simulink model "Discrete_Domain"  (R2020a)
settings: Solver=VariableStepAuto  StartTime=0.0  StopTime=20  RelTol=1e-3
libraries: cstblocks x18
settings Model: Creator=Tayla  LastModifiedBy=Tayla
settings SolverCC: AlgebraicLoopSolver=LineSearch
settings DebuggingCC: AlgebraicLoopMsg=none
settings ConfigComp: PLC_TargetIDE=codesys23

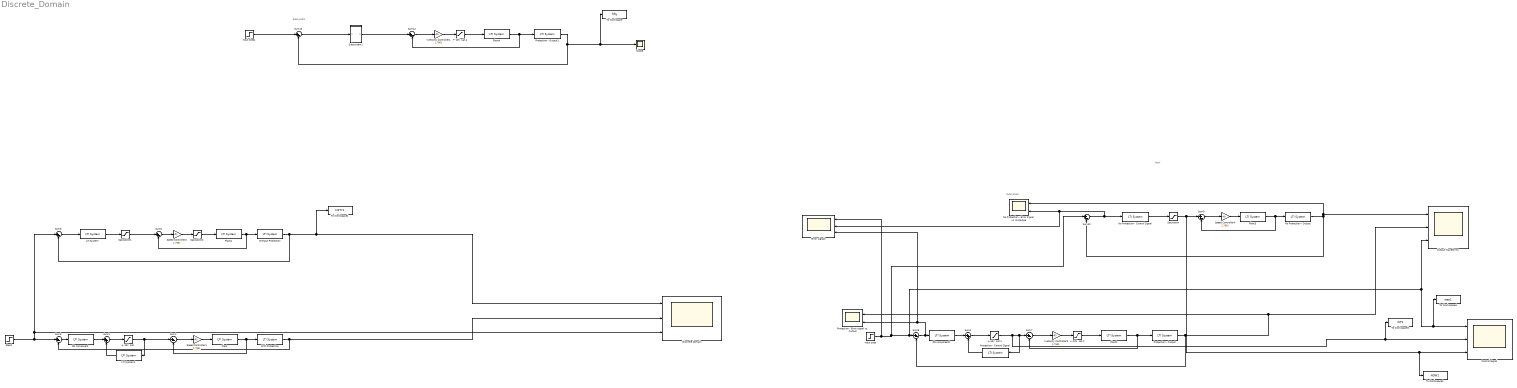
== system Discrete_Domain ==
  note: NoW
  note: Subsystem
  note: Subsystem
  " Protection - Output" : cstblocks/LTI System  sys=effectsD  IC=[]
  " Protection - Output1" : cstblocks/LTI System  sys=effectsD  IC=[]
  +-10V  sat.{,1..2,4} (4 alike) : Saturate  UpperLimit=10  LowerLimit=-10  LinearizeAsGain=off  ZeroCross=off
  Control Signal : Scope  NumInputPorts=3
  Discrete Domain : Scope  NumInputPorts=3
  Error signals : Scope  NumInputPorts=3
  Input step : Step  Time=0  After=2.61  SampleTime=0
  Input step1 : Step  After=4.35  SampleTime=0
  LTI System : cstblocks/LTI System  sys=Pos_HPF_2_Dis  IC=[]
  LTI System1 : cstblocks/LTI System  sys=PI_Dis  IC=[]
  No Protection - Control Signal : cstblocks/LTI System  sys=Pos_HPF_2_Dis  IC=[]
  No Protection - Error signal vs. Outputpe : Scope  NumInputPorts=2
  No Protection - Output : cstblocks/LTI System  sys=effectsD  IC=[]
  Output Waveforms : Scope  NumInputPorts=3
  PD component : cstblocks/LTI System  sys=Kp_Dis  IC=[]
  PD component1 : cstblocks/LTI System  sys=Kp_Dis  IC=[]
  Plant : cstblocks/LTI System  sys=tf_2  IC=[]
  Plant{1..4} (4 alike) : cstblocks/LTI System  sys=tf_1  IC=[]
  Protection - Control Signal : cstblocks/LTI System  sys=PI_Dis  IC=[]
  Protection - Error signal vs. Output : Scope  NumInputPorts=2
  Saturation : Saturate  UpperLimit=10  LowerLimit=-10
  Saturation1 : Saturate  UpperLimit=10  LowerLimit=-10
  Saturation2 : Saturate  UpperLimit=10  LowerLimit=-10
  Scope : Scope
  Speed Controller1 : Gain  Gain=1.7961
  Speed Controller2 : Gain  Gain=1.7961
  Speed Controller4 : Gain  Gain=1.7961
  Step1 : Step  After=4.35  SampleTime=0.15
  Subsystem1 : Subsystem  TreatAsAtomicUnit=on  SystemSampleTime=0.15
  Sum1 : Sum  Inputs=|++
  Sum{2..3,5..10,12..13} (10 alike) : Sum  Inputs=|+-
  Sum4 : Sum  Inputs=|++
  To Workspace : ToWorkspace  VariableName=fifty  SaveFormat=Timeseries  SampleTime=0.15
  To Workspace1 : ToWorkspace  VariableName=FIFTY1  SaveFormat=Timeseries  SampleTime=-1
  To Workspace2 : ToWorkspace  VariableName=NOW1  SaveFormat=Timeseries  SampleTime=0.15
  To Workspace3 : ToWorkspace  VariableName=WP1  SaveFormat=Timeseries  SampleTime=0.15
  To Workspace4 : ToWorkspace  VariableName=step1  SaveFormat=Timeseries  SampleTime=0.15
  Vvelocity Controller1 : Gain  Gain=1.7961
  Vvelocity Controller3 : Gain  Gain=1.7961
  With Protection : cstblocks/LTI System  sys=effectsD  IC=[]
  Without Protection : cstblocks/LTI System  sys=effectsD  IC=[]
  wires:
  Speed Controller1/1 -> Plant/1
  Sum3/1 -> PD component/1
  Plant/1 -> Sum2/2, With Protection/1
  With Protection/1 -> Sum3/2, Discrete Domain/2
  Sum2/1 -> Speed Controller1/1
  +-10V  sat./1 -> Sum2/1, LTI System1/1
  Sum1/1 -> +-10V  sat./1
  LTI System1/1 -> Sum1/2
  PD component/1 -> Sum1/1
  Sum5/1 -> Speed Controller2/1
  Step1/1 -> Discrete Domain/3, Sum6/1, Sum3/1
  Speed Controller2/1 -> Saturation2/1
  Without Protection/1 -> To Workspace1/1, Discrete Domain/1, Sum6/2
  Plant1/1 -> Sum5/2, Without Protection/1
  Sum6/1 -> LTI System/1
  LTI System/1 -> Saturation1/1
  Sum7/1 -> Vvelocity Controller3/1
  Sum4/1 -> +-10V  sat.1/1
  PD component1/1 -> Sum4/1
  +-10V  sat.1/1 -> To Workspace3/1, Control Signal/2, Sum7/1, Protection - Control Signal/1
  Sum8/1 -> Error signals/3, Protection - Error signal vs. Output/2, PD component1/1
  Plant2/1 -> " Protection - Output"/1, Sum7/2
  " Protection - Output"/1 -> Output Waveforms/2, Protection - Error signal vs. Output/1, Sum8/2
  Protection - Control Signal/1 -> Sum4/2
  Saturation1/1 -> Sum5/1
  +-10V  sat.2/1 -> Plant2/1
  Vvelocity Controller3/1 -> +-10V  sat.2/1
  No Protection - Output/1 -> No Protection - Error signal vs. Outputpe/1, Output Waveforms/1, Sum10/2
  No Protection - Control Signal/1 -> Saturation/1
  Input step/1 -> Error signals/1, Sum10/1, To Workspace4/1, Control Signal/1, Output Waveforms/3, Sum8/1
  Saturation/1 -> To Workspace2/1, Control Signal/3, Sum9/1
  Sum9/1 -> Speed Controller4/1
  Speed Controller4/1 -> Plant3/1
  Plant3/1 -> Sum9/2, No Protection - Output/1
  " Protection - Output1"/1 -> To Workspace/1, Scope/1, Sum13/2
  Subsystem1/1(Out1) -> Sum12/1
  Sum13/1 -> Subsystem1/1(In1)
  Input step1/1 -> Sum13/1
  Sum12/1 -> Vvelocity Controller1/1
  +-10V  sat.4/1 -> Plant4/1
  Plant4/1 -> " Protection - Output1"/1, Sum12/2
  Vvelocity Controller1/1 -> +-10V  sat.4/1
  Saturation2/1 -> Plant1/1
  Sum10/1 -> Error signals/2, No Protection - Error signal vs. Outputpe/2, No Protection - Control Signal/1

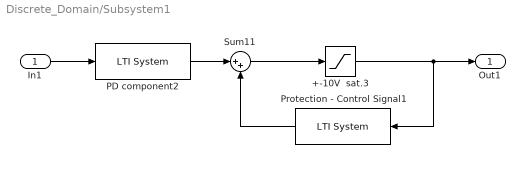
== system Discrete_Domain/Subsystem1 ==
  In1 : Inport
  +-10V  sat.3 : Saturate  UpperLimit=10  LowerLimit=-10  LinearizeAsGain=off  ZeroCross=off
  PD component2 : cstblocks/LTI System  sys=Kp_Dis  IC=[]
  Protection - Control Signal1 : cstblocks/LTI System  sys=PI_Dis  IC=[]
  Sum11 : Sum  Inputs=|++
  Out1 : Outport
  wires:
  PD component2/1 -> Sum11/1
  +-10V  sat.3/1 -> Out1/1, Protection - Control Signal1/1
  Protection - Control Signal1/1 -> Sum11/2
  In1/1 -> PD component2/1
  Sum11/1 -> +-10V  sat.3/1
